simulink model "LiDARReadVelocity"  (Simulink 7.9)
settings: Solver=ode3  StartTime=0.0  StopTime=inf  FixedStep=.05  RelTol=1e-3
libraries: realtime_pacer_lib x1
settings Model: Creator=ipainter  LastModifiedBy=TCA
settings DebuggingCC: SolverPrmCheckMsg=none
settings GRTTargetCC: CombineOutputUpdateFcns=off  GRTInterface=on

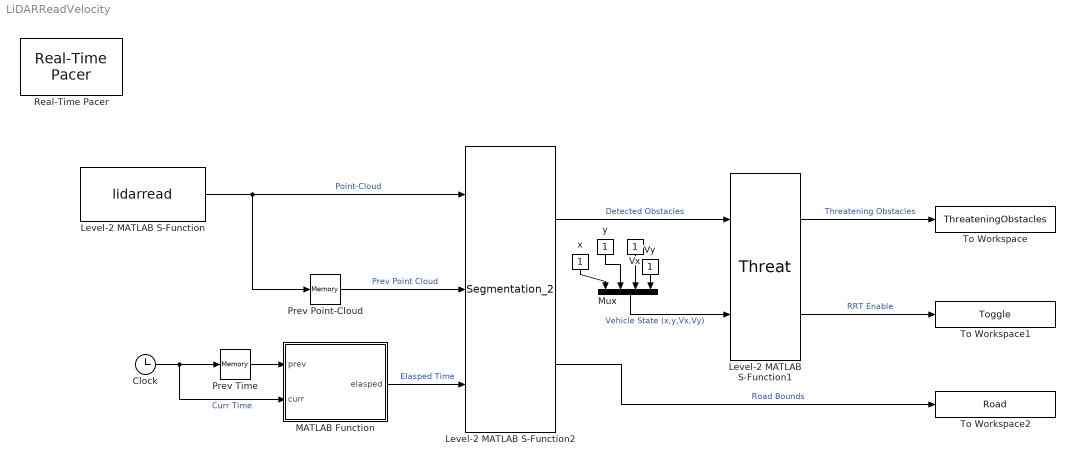
== system LiDARReadVelocity ==
  Clock : Clock
  Level-2 MATLAB S-Function : M-S-Function  FunctionName=lidarread
  Level-2 MATLAB S-Function1 : M-S-Function  FunctionName=Threat  Parameters=1
  Level-2 MATLAB S-Function2 : M-S-Function  FunctionName=Segmentation_2  Parameters=15,13,1
  MATLAB Function : MATLAB Function  TreatAsAtomicUnit=on
  Mux : Mux
  Prev Point-Cloud : Memory
  Prev Time : Memory
  Real-Time Pacer : realtime_pacer_lib/Real-Time Pacer  simTimePerRealTime=1
  To Workspace : ToWorkspace  VariableName=ThreateningObstacles  SampleTime=-1  SaveFormat=Structure With Time
  To Workspace1 : ToWorkspace  VariableName=Toggle  SampleTime=-1  SaveFormat=Structure With Time
  To Workspace2 : ToWorkspace  VariableName=Road  SampleTime=-1  SaveFormat=Structure With Time
  Vx : Constant
  Vy : Constant
  x : Constant
  y : Constant
  wires:
  Level-2 MATLAB S-Function2/1 -> Level-2 MATLAB S-Function1/1  "Detected Obstacles"
  Level-2 MATLAB S-Function/1 -> Prev Point-Cloud/1, Level-2 MATLAB S-Function2/1  "Point-Cloud"
  Prev Point-Cloud/1 -> Level-2 MATLAB S-Function2/2  "Prev Point Cloud"
  Clock/1 -> MATLAB Function/2(curr), Prev Time/1  "Curr Time"
  Prev Time/1 -> MATLAB Function/1(prev)
  MATLAB Function/1(elasped) -> Level-2 MATLAB S-Function2/3  "Elasped Time"
  Level-2 MATLAB S-Function2/2 -> To Workspace2/1  "Road Bounds"
  Level-2 MATLAB S-Function1/1 -> To Workspace/1  "Threatening Obstacles"
  Mux/1 -> Level-2 MATLAB S-Function1/2  "Vehicle State (x,y,Vx,Vy)"
  Level-2 MATLAB S-Function1/2 -> To Workspace1/1  "RRT Enable"
  x/1 -> Mux/1
  y/1 -> Mux/2
  Vx/1 -> Mux/3
  Vy/1 -> Mux/4

== matlab function MATLAB Function ==
  data: prev input double; elasped output double; curr input double
function elasped = fcn(prev,curr)
%#codegen

elasped = curr-prev;
